simulink model "HybridPowertrain_TestBench_Final"  (R2017a)
settings: Solver=ode1  StartTime=0.0  StopTime=1400  FixedStep=0.01  RelTol=1e-3  EnableMultiTasking=on
undefined symbols (not defined in the file): AccActPos, air, Atm_temp, bms_inletair_temp, BMS_IstStrom, bms_maxchargecurrent, bms_maxdischargecurrent, BMS_Notfallkuehlung, BMS_SOC, BrkPdlPos, cal, Cells, Chg, D1_Commanded_Torque, D1_DC_Bus_Voltage, D2_Motor_Speed, D2_Torque_Feedback, DriverControls, EcoCAR3_Lib, Em, EngActStdyStTorq, Engine, EngSpd, env, ESS, fd, g, gb, Gearbox, GearBox, gps_lat, gps_long, Grade, I_loss, IMG, InstFuelConsmpRate, KeyPosition, lib_ESS_plant_V1_2, Loss, max_vehicle_rad_air_flow, mot, mph2kph, mph2ms, NeutralGear, ParkGear, PPEI_Engine_General_Status_2__ThrPos, PTEI_Engine_Torque_Status__EngActStdyStTorq, R_0, R_1, Ratio, RegenBrkDisable, rho, SampleTime, ShiftLeverPosition, SOC_bp, SOC_init, Spd, Speed, SW_CS_ON, SW_Engine_ON ... (+15)
libraries: simulink x39, fl_lib x13, nesl_utility x8, Utility x1, EC2_libraries x1
(part 1 of 5)
settings Model: Creator=Sajjan  LastModifiedBy=vraj
settings SolverCC: ZeroCrossAlgorithm=Adaptive
settings DataIOCC: LimitDataPoints=on  SaveFormat=Array
settings OptimizationCC: LifeSpan=inf
settings DebuggingCC: SFUnexpectedBacktrackingDiag=warning  SFNoUnconditionalDefaultTransitionDiag=warning  SFExecutionAtInitializationDiag=none
settings HardwareCC: ProdBitPerPointer=32  ProdBitPerSizeT=32  ProdBitPerPtrDiffT=32  ProdLargestAtomicFloat=None  ProdIntDivRoundTo=Undefined  ProdEndianess=Unspecified  ProdWordSize=32  ProdHWDeviceType=32-bit Generic
settings ModelReferenceCC: PropagateSignalLabelsOutOfModel=off
settings GRTTargetCC: TargetLangStandard=C89/C90 (ANSI)  GeneratePreprocessorConditionals=Disable all
settings ConfigComp: CovMetricSettings=dw  CovHtmlReporting=on  CovSaveCumulativeToWorkspaceVar=on  CovSaveSingleToWorkspaceVar=on  CovExternalEMLEnable=off

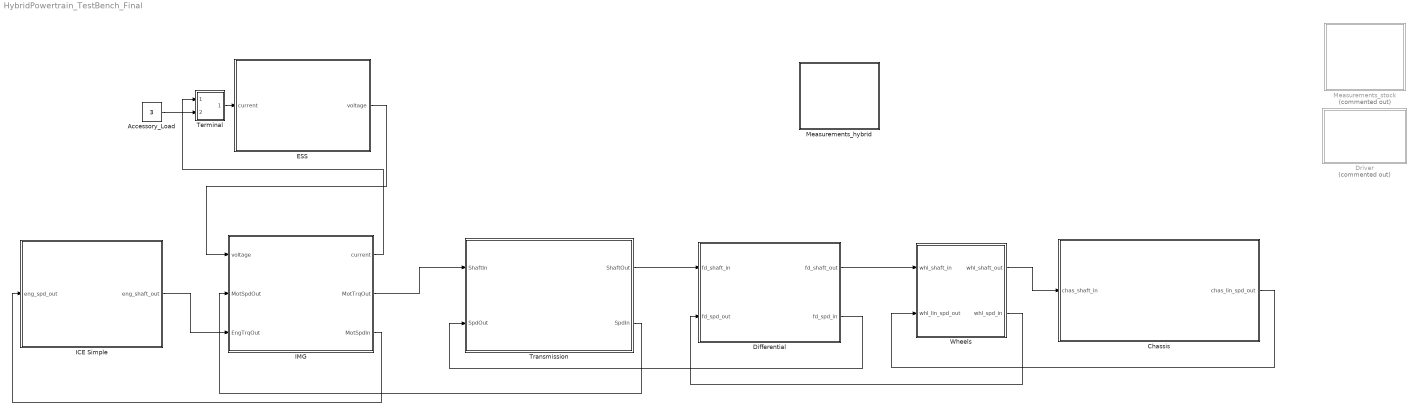
== system HybridPowertrain_TestBench_Final ==
  Accessory_Load : Constant  Value=3
  Chassis : Subsystem  AncestorBlock=Chassis/Chassis
      mask Display:
      | image('/media/vraj/Matlab/Workspace/EcoCAR3/MIL_Code/P2_PHEV_MIL_EC3Y4_V1/Images/Chassis.JPG');
      | color('red');
      | port_label('input',1,'ShaftIn');
      | port_label('output',1,'SpdOut');
  Differential : Subsystem  AncestorBlock=Differential/Differential
      mask Display:
      | image('Images/Diff.jpg');
      | color('red');
      | port_label('input',1,'ShaftIn')
      | port_label('input',2,'SpdOut')
      | port_label('output',1,'ShaftOut')
      | port_label('output',2,'SpdIn')
  Driver : Subsystem  Commented=on
      mask Display: image('Images\Driver.jpg')
  ESS : Subsystem  AncestorBlock=lib_ESS_plant_V1_2/ESS
      mask Display:
      | image('/media/vraj/Matlab/Workspace/EcoCAR3/MIL_Code/P2_PHEV_MIL_EC3Y4_V1/Images/ESS.jpg')
      | color('red');
      | port_label('Input',1,'Crr');
      | port_label('Output',1,'Volt');
  ICE Simple : Subsystem  AncestorBlock=Engine_simple/ICE Simple
      mask Display:
      | image(imread('EngineTopLevel.jpg'),'center')
      | color('red');
      | port_label('input',1,'SpdOut')
      | port_label('output',1,'ShaftOut')
  IMG : Subsystem  AncestorBlock=IMG/IMG
      mask Display:
      | image(imread('motor.png'),'center')
      | color('red');
      | port_label('Input',1,'Volt');
      | port_label('Input',2,'MotSpdOut');
      | port_label('Output',1,'Crr');
      | port_label('Output',2,'MotTrqOut');
      | port_label('Output',3,'MotSpdIn');
  Measurements_hybrid : Subsystem
  Measurements_stock : Subsystem  Commented=on
  Terminal : Subsystem
  Transmission : Subsystem  AncestorBlock=Transmission/Transmission
      mask Display:
      | image('/media/vraj/Matlab/Workspace/EcoCAR3/MIL_Code/P2_PHEV_MIL_EC3Y4_V1/Images/Trans.PNG')
      | color('red');
      | port_label('Input',1,'ShaftIn')
      | port_label('Input',2,'SpdOut')
      | port_label('Output',1,'ShaftOut')
      | port_label('Output',2,'SpdIn')
  Wheels : Subsystem  AncestorBlock=Wheels/Wheels
      mask Display:
      | image('Images/Wheel.jpg');
      | color('red');
      | port_label('input',1,'ShaftIn');
      | port_label('input',2,'SpdOut');
      | port_label('output',1,'ShaftOut');
      | port_label('output',2,'SpdIn');
  wires:
  Differential/1(fd_shaft_out) -> Wheels/1(whl_shaft_in)
  Wheels/1(whl_shaft_out) -> Chassis/1(chas_shaft_in)
  Chassis/1(chas_lin_spd_out) -> Wheels/2(whl_lin_spd_out)
  Differential/2(fd_spd_in) -> Transmission/2(SpdOut)
  Transmission/1(ShaftOut) -> Differential/1(fd_shaft_in)
  Transmission/2(SpdIn) -> IMG/2(MotSpdOut)
  Wheels/2(whl_spd_in) -> Differential/2(fd_spd_out)
  IMG/3(MotSpdIn) -> ICE Simple/1(eng_spd_out)
  ESS/1(voltage) -> IMG/1(voltage)
  Terminal/1(Out1) -> ESS/1(current)
  Accessory_Load/1 -> Terminal/2(In2)
  IMG/2(MotTrqOut) -> Transmission/1(ShaftIn)
  ICE Simple/1(eng_shaft_out) -> IMG/3(EngTrqOut)
  IMG/1(current) -> Terminal/1(In1)

== system HybridPowertrain_TestBench_Final/Chassis ==
  note: Total opposing
      | force (N)
  chas_shaft_in : Inport
  >1 : Saturate  UpperLimit=inf  LowerLimit=0
  Bus Selector : BusSelector  OutputSignals=veh_grade_force_simu,drag force
  Bus Selector1 : BusSelector  OutputSignals=whl_force_out_simu,whl_mass_out_simu
  Clock : Clock
  Driver Interface : Subsystem
  Grade : Lookup  InputValues=time  Table=Grade
  Soft BCM : Subsystem
      mask Display: image('SoftECU.jpg')
  Sum2 : Sum  Inputs=|++  SaturateOnIntegerOverflow=on  InputSameDT=on  OutDataTypeStr=Inherit: Same as first input
  Sum3 : Sum  Inputs=-+  SaturateOnIntegerOverflow=on  InputSameDT=on  OutDataTypeStr=Inherit: Same as first input
  To Workspace1 : ToWorkspace  VariableName=distance_miles_hist  SampleTime=-1
      settings: Decimation=WORKSPACE_DECIMATION
  To Workspace2 : ToWorkspace  VariableName=veh_dist_meter_hist  SampleTime=-1
      settings: Decimation=WORKSPACE_DECIMATION
  To Workspace3 : ToWorkspace  VariableName=veh_spd_mps_hist  SampleTime=-1
      settings: Decimation=WORKSPACE_DECIMATION
  To Workspace7 : ToWorkspace  VariableName=veh_spd_mph_hist  SampleTime=-1
      settings: Decimation=WORKSPACE_DECIMATION
  Velocity1 : Integrator  LimitOutput=on  LowerSaturationLimit=0
  Velocity2 : Integrator  LimitOutput=on  LowerSaturationLimit=0
  m to miles : Gain  Gain=0.00062
  m to miles1 : Gain  Gain=1/1000
  m/s to kph : Gain  Gain=3.6
  ms to mph : Gain  Gain=1/mph2ms
  non-zero division1 : Subsystem
      mask Display: disp('divider \n I1/I2')
  vehicle losses : Subsystem
  vehicle total mass : Constant  Value=veh.init.mass
  chas_lin_spd_out : Outport
  tag scope: BCM_to_HCU=global, chas_plant_force_in=global, chas_plant_force_loss=global, chas_plant_grade=global, chas_plant_lin_accel=global, chas_plant_lin_spd_out=global, chas_plant_mass=global, chas_plant_mass_static=global, veh_dist_km=global, veh_dist_miles=global
  wires:
  Grade/1 -> vehicle losses/2(Road grade), [chas_plant_grade]
  Bus Selector/2 -> [chas_plant_force_loss]  "<drag force>"
  Bus Selector/1 -> [chas_plant_force_grade]  "<veh_grade_force_simu>"
  vehicle total mass/1 -> Sum2/1, [chas_plant_mass_static]
  Velocity1/1 -> vehicle losses/1(veh spd simu), m/s to kph/1, Velocity2/1, To Workspace3/1, ms to mph/1, chas_lin_spd_out/1
  non-zero division1/1(Out1) -> Velocity1/1, [chas_plant_lin_accel]
  Sum3/1 -> non-zero division1/1(In1)
  Sum2/1 -> non-zero division1/2(In2), [chas_plant_mass]
  >1/1 -> Sum2/2
  Bus Selector1/2 -> >1/1  "<whl_mass_out_simu>"
  Bus Selector1/1 -> [chas_plant_force_in], Sum3/2  "<whl_force_out_simu>"
  chas_shaft_in/1 -> Bus Selector1/1
  vehicle losses/1(info) -> Bus Selector/1
  Soft BCM/1(Out1) -> [BCM_to_HCU]
  m/s to kph/1 -> [chas_plant_lin_spd_out]
  ms to mph/1 -> To Workspace7/1
  Clock/1 -> Grade/1
  Velocity2/1 -> To Workspace2/1, m to miles1/1, m to miles/1
  m to miles/1 -> [veh_dist_miles], To Workspace1/1
  m to miles1/1 -> [veh_dist_km]
  vehicle losses/2(veh_force_loss_simu) -> Sum3/1

== system HybridPowertrain_TestBench_Final/Differential ==
  fd_shaft_in : Inport
  fd_spd_out : Inport  Port=2
  Bus Creator : BusCreator  Inputs=2
  Bus Selector : BusSelector  OutputSignals=gb_trq_out,gb_inertia_out
  Inertia calculation : Subsystem
  Speed calculation : Subsystem
  Torque calculation : Subsystem
  fd_shaft_out : Outport
  fd_spd_in : Outport  Port=2
  wires:
  Torque calculation/1(trq out) -> Bus Creator/1  "fd_trq_out_simu"
  fd_spd_out/1 -> Speed calculation/1(spd out)
  Speed calculation/1(spd in) -> Torque calculation/1(spd in), fd_spd_in/1
  Inertia calculation/1(inertia out) -> Bus Creator/2  "fd_inertia_out_simu"
  Bus Selector/1 -> Torque calculation/2(trq in)  "<gb_trq_out>"
  Bus Selector/2 -> Inertia calculation/1(inertia in)  "<gb_inertia_out>"
  fd_shaft_in/1 -> Bus Selector/1
  Bus Creator/1 -> fd_shaft_out/1

== system HybridPowertrain_TestBench_Final/Driver ==
  Bus Creator : BusCreator  Inputs=10
  Bus Selector : BusSelector  OutputSignals=GFD_Light,HV_Chg_Light,Veh_Ready_Light
  Constant : Constant  Commented=on  Value=0
  Display : Display
  Display1 : Display
  Display2 : Display
  Driver Control : Subsystem
  Manual Control : Subsystem  Commented=on
  Multiport Switch1 : MultiPortSwitch  Commented=on  DataPortOrder=Zero-based contiguous  Inputs=2
  Subsystem : Subsystem
  tag scope: Driver_Request=global
  wires:
  Driver Control/1(Key Position) -> Bus Creator/1  "KeyPos"
  Driver Control/2(APP[%]) -> Subsystem/1(In1)  "drv_APP_req_[%]"
  Driver Control/3(BPP[%]) -> Bus Creator/4  "drv_BPP_req_[%]"
  Driver Control/4(Shift Lever Position) -> Bus Creator/5  "ShiftLvrPos"
  Driver Control/5(EVSE_Pluggin) -> Bus Creator/6  "EVSE_Plugged"
  Constant/1 -> Multiport Switch1/1
  Manual Control/1(Out1) -> Multiport Switch1/3
  Bus Creator/1 -> [Driver_Request]
  Driver Control/6(Veh_Spd) -> Bus Creator/7  "Veh_Spd"
  Driver Control/7(Regen_Disable) -> Bus Creator/8  "SW_Regen_Disable"
  Driver Control/8(Engine_On) -> Bus Creator/9  "SW_Engine_ON"
  Driver Control/9(CS_On) -> Bus Creator/10  "SW_CS_ON"
  [Digital] -> Bus Selector/1
  Bus Selector/1 -> Display/1  "<GFD_Light>"
  Bus Selector/2 -> Display1/1  "<HV_Chg_Light>"
  Bus Selector/3 -> Display2/1  "<Veh_Ready_Light>"
  Subsystem/1(APP1) -> Bus Creator/2
  Subsystem/2(APP2) -> Bus Creator/3

== system HybridPowertrain_TestBench_Final/ESS ==
  note: BMS_to_Actuators
  current : Inport
  ESS : Subsystem
      mask Display:
      | image('/media/vraj/Matlab/Workspace/EcoCAR3/MIL_Code/P2_PHEV_MIL_EC3Y4_V1/Images/ESS.jpg')
      | color('red');
      | port_label('Input',2,'Crr');
      | port_label('Output',2,'Volt');
  Inputs : Subsystem  AncestorBlock=lib_DCDC/DC-DC Converter/Inputs
  Outputs : Subsystem
  Soft BMS : Subsystem  RequirementInfo={} %GIDa_f148d73b_346e_4e28_9569_8b82e4a6609c
      mask Display: image('/media/vraj/Matlab/Workspace/EcoCAR3/MIL_Code/P2_PHEV_MIL_EC3Y4_V1/Images/SoftECU.jpg')
  voltage : Outport
  wires:
  current/1 -> ESS/2("Crr ")
  Soft BMS/2(Output2) -> ESS/1("In ")
  ESS/1(out) -> Soft BMS/2(Input2)  "Sensors_to_BMS"
  ESS/2(Voltage) -> voltage/1
  Soft BMS/1(CAN) -> Outputs/1(Outputs)
  Inputs/1(Inputs) -> Soft BMS/1(Input1)

== system HybridPowertrain_TestBench_Final/ICE Simple ==
  eng_spd_out : Inport
  Engine Plant Modified : Subsystem
      mask Display:
      | image(imread('EngineTopLevel.jpg'),'center')
      | color('red');
      | port_label('input',2,'SpdOut')
      | port_label('output',2,'ShaftOut')
  Inputs : Subsystem
  Soft ECM : Subsystem
      mask Display: image('SoftECU.jpg')
  eng_shaft_out : Outport
  tag scope: ECM_to_HCU=global
  wires:
  Engine Plant Modified/2(eng_shaft_out) -> eng_shaft_out/1
  eng_spd_out/1 -> Engine Plant Modified/2(eng_spd_out)
  Soft ECM/2(Out1) -> Engine Plant Modified/1("In ")  "ECM_to_Actuators"
  Inputs/1(Inputs) -> Soft ECM/1(In)
  Soft ECM/1(Out) -> [ECM_to_HCU]
  Engine Plant Modified/1(Out) -> Soft ECM/2(In1)

== system HybridPowertrain_TestBench_Final/IMG ==
  voltage : Inport
  MotSpdOut : Inport  Port=2
  EngTrqOut : Inport  Port=3
  IMG Plant : Subsystem
      mask Display:
      | image('/media/vraj/Matlab/Workspace/EcoCAR3/MIL_Code/P2_PHEV_MIL_EC3Y4_V1/Images/motor.png')
      | color('red');
      | port_label('Input',2,'Volt');
      | port_label('Input',3,'SpdOut');
      | port_label('Input',1,'MCU_cmd');
      | port_label('Output',1,'Sensor_Out');
      | port_label('Output',2,'Crr');
      | port_label('Output',3,'MotTrqOut');
      | port_label('Output',4,'MotSpdIn');
  Soft MCU : Subsystem
      mask Display: image('/media/vraj/Matlab/Workspace/EcoCAR3/MIL_Code/P2_PHEV_MIL_EC3Y4_V1/Images/SoftECU.jpg')
  current : Outport
  MotTrqOut : Outport  Port=2
  MotSpdIn : Outport  Port=3
  tag scope: MCU_to_HCU=global
  wires:
  IMG Plant/1(Out1) -> Soft MCU/2(In1)  "Sensors_to_MCU"
  Soft MCU/2(Out1) -> IMG Plant/1("In1 ")  "MCU_to_Actuators"
  Soft MCU/1(Out) -> [MCU_to_HCU]
  [HCU_to_HV_CAN] -> Soft MCU/1(In)
  IMG Plant/2(current) -> current/1
  voltage/1 -> IMG Plant/2(voltage)
  IMG Plant/3(MotTrqOut) -> MotTrqOut/1
  MotSpdOut/1 -> IMG Plant/3(SpdOut)
  IMG Plant/4(MotSpdIn) -> MotSpdIn/1
  EngTrqOut/1 -> IMG Plant/4(EngTrqOut)

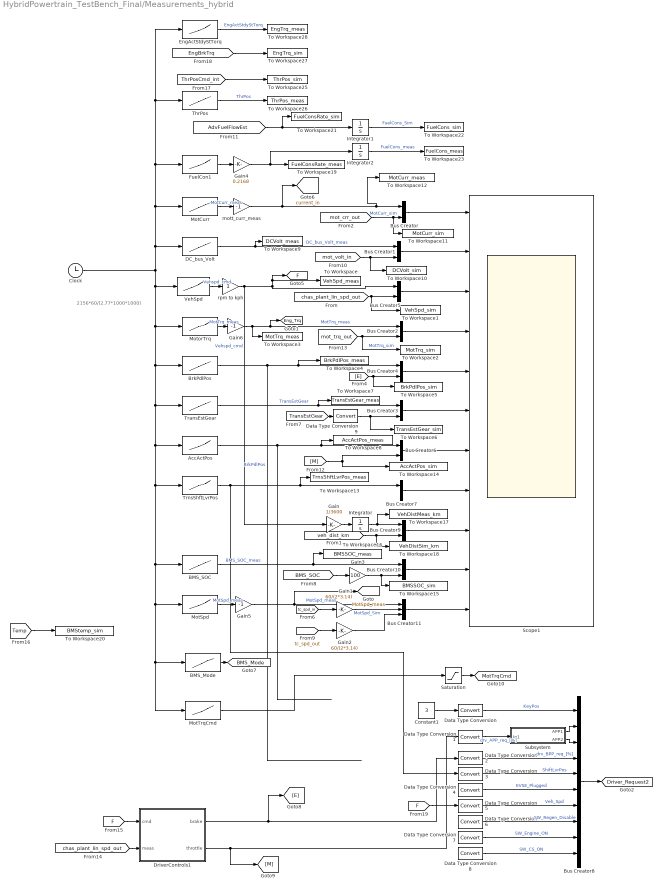
== system HybridPowertrain_TestBench_Final/Measurements_hybrid ==
  note: 2156*60/(2.77*1000*1000)
  AccActPos : Lookup  InputValues=Times  Table=AccActPos
  BMS_Mode : Lookup  InputValues=[0 0.9 1 2 3]  Table=[0 0 1 1 1]
  BMS_SOC : Lookup  InputValues=Times  Table=BMS_SOC
  BrkPdlPos : Lookup  InputValues=Times  Table=BrkPdlPos
  Bus Creator{,1..7,9..10} (10 alike) : BusCreator  Inputs=2
  Bus Creator11 : BusCreator  Inputs=3
  Bus Creator8 : BusCreator  Inputs=10
  Clock : Clock
  Constant1 : Constant  Value=3
  DC_bus_Volt : Lookup  InputValues=Times  Table=D1_DC_Bus_Voltage
  Data Type Conversion{,1..9} (10 alike) : DataTypeConversion
  DriverControls1 : Subsystem  AncestorBlock=EcoCAR3_Lib/DriverControls
  EngActStdyStTorq : Lookup  InputValues=Times  Table=EngActStdyStTorq
  FuelCon1 : Lookup  InputValues=Times  Table=InstFuelConsmpRate
  Gain : Gain  Gain=1/3600
  Gain1 : Gain  Gain=60/(2*3.14)
  Gain2 : Gain  Gain=60/(2*3.14)
  Gain3 : Gain  Gain=100
  Gain4 : Gain  Gain=0.2168
  Gain5 : Gain  Gain=-1
  Gain6 : Gain  Gain=-1
  Integrator : Integrator
  Integrator1 : Integrator
  Integrator2 : Integrator
  MotCurr : Lookup  InputValues=Times  Table=BMS_IstStrom
  MotSpd : Lookup  InputValues=Times  Table=D2_Motor_Speed
  MotTrqCmd : Lookup  InputValues=Times  Table=D1_Commanded_Torque
  MotorTrq : Lookup  InputValues=Times  Table=D2_Torque_Feedback
  Saturation : Saturate  UpperLimit=150  LowerLimit=0
  Scope1 : Scope  NumInputPorts=11
  Subsystem : Subsystem
  ThrPos : Lookup  InputValues=Times  Table=ThrPos
  To Workspace : ToWorkspace  VariableName=VehSpd_meas  SaveFormat=Timeseries  SampleTime=-1
  To Workspace1 : ToWorkspace  VariableName=VehSpd_sim  SaveFormat=Timeseries  SampleTime=-1
  To Workspace10 : ToWorkspace  VariableName=DCVolt_sim  SaveFormat=Timeseries  SampleTime=-1
  To Workspace11 : ToWorkspace  VariableName=MotCurr_sim  SaveFormat=Timeseries  SampleTime=-1
  To Workspace12 : ToWorkspace  VariableName=MotCurr_meas  SaveFormat=Timeseries  SampleTime=-1
  To Workspace13 : ToWorkspace  VariableName=TrnsShftLvrPos_meas  SaveFormat=Timeseries  SampleTime=-1
  To Workspace14 : ToWorkspace  VariableName=AccActPos_sim  SaveFormat=Timeseries  SampleTime=-1
  To Workspace15 : ToWorkspace  VariableName=BMSSOC_sim  SaveFormat=Timeseries  SampleTime=-1
  To Workspace16 : ToWorkspace  VariableName=BMSSOC_meas  SaveFormat=Timeseries  SampleTime=-1
  To Workspace17 : ToWorkspace  VariableName=VehDistMeas_km  SaveFormat=Timeseries  SampleTime=-1
  To Workspace18 : ToWorkspace  VariableName=VehDistSim_km  SaveFormat=Timeseries  SampleTime=-1
  To Workspace19 : ToWorkspace  VariableName=FuelConsRate_meas  SaveFormat=Timeseries  SampleTime=-1
  To Workspace2 : ToWorkspace  VariableName=MotTrq_sim  SaveFormat=Timeseries  SampleTime=-1
  To Workspace20 : ToWorkspace  VariableName=BMStemp_sim  SaveFormat=Timeseries  SampleTime=-1
  To Workspace21 : ToWorkspace  VariableName=FuelConsRate_sim  SaveFormat=Timeseries  SampleTime=-1
  To Workspace22 : ToWorkspace  VariableName=FuelCons_sim  SaveFormat=Timeseries  SampleTime=-1
  To Workspace23 : ToWorkspace  VariableName=FuelCons_meas  SaveFormat=Timeseries  SampleTime=-1
  To Workspace25 : ToWorkspace  VariableName=ThrPos_sim  SaveFormat=Timeseries  SampleTime=-1
  To Workspace26 : ToWorkspace  VariableName=ThrPos_meas  SaveFormat=Timeseries  SampleTime=-1
  To Workspace27 : ToWorkspace  VariableName=EngTrq_sim  SaveFormat=Timeseries  SampleTime=-1
  To Workspace28 : ToWorkspace  VariableName=EngTrq_meas  SaveFormat=Timeseries  SampleTime=-1
  To Workspace3 : ToWorkspace  VariableName=MotTrq_meas  SaveFormat=Timeseries  SampleTime=-1
  To Workspace4 : ToWorkspace  VariableName=BrkPdlPos_meas  SaveFormat=Timeseries  SampleTime=-1
  To Workspace5 : ToWorkspace  VariableName=BrkPdlPos_sim  SaveFormat=Timeseries  SampleTime=-1
  To Workspace6 : ToWorkspace  VariableName=TransEstGear_sim  SaveFormat=Timeseries  SampleTime=-1
  To Workspace7 : ToWorkspace  VariableName=TransEstGear_meas  SaveFormat=Timeseries  SampleTime=-1
  To Workspace8 : ToWorkspace  VariableName=AccActPos_meas  SaveFormat=Timeseries  SampleTime=-1
  To Workspace9 : ToWorkspace  VariableName=DCVolt_meas  SaveFormat=Timeseries  SampleTime=-1
  TransEstGear : Lookup  InputValues=Times  Table=TransEstGear
  TrnsShftLvrPos : Lookup  InputValues=Times  Table=TrnsShftLvrPos
  VehSpd : Lookup_n-D  NumberOfTableDimensions=1  BreakpointsForDimension1=Times  Table=WhlGrndVlctyRtDrvn  InternalRulePriority=Speed  RndMeth=Simplest  InputSameDT=on
  mott_curr_meas : Gain  Gain=-1
  rpm to kph : Gain
  tag scope: BMS_Mode=global, Driver_Request2=global, Eng_Trq=global, F=global, MotSpd_meas=global, MotTrqCmd=global, current_in=global
  wires:
  Gain2/1 -> Bus Creator11/3
  [tc_spd_out] -> Gain2/1
  Gain1/1 -> Bus Creator11/2  "MotSpd_Sim"
  Bus Creator11/1 -> Scope1/11
  [tc_spd_in] -> Gain1/1
  Gain5/1 -> [MotSpd_meas], Bus Creator11/1  "MotSpd_meas"
  Bus Creator10/1 -> Scope1/10
  Gain/1 -> Integrator/1
  Bus Creator9/1 -> Scope1/9
  Integrator/1 -> To Workspace17/1, Bus Creator9/1
  [veh_dist_km] -> Bus Creator9/2, To Workspace18/1
  [M] -> Bus Creator6/2, To Workspace14/1
  Data Type Conversion9/1 -> To Workspace6/1, Bus Creator3/2
  [F] -> Data Type Conversion5/1
  Constant1/1 -> Data Type Conversion/1
  Subsystem/2(APP2) -> Bus Creator8/3
  Subsystem/1(APP1) -> Bus Creator8/2
  Data Type Conversion8/1 -> Bus Creator8/10  "SW_CS_ON"
  Data Type Conversion7/1 -> Bus Creator8/9  "SW_Engine_ON"
  Data Type Conversion6/1 -> Bus Creator8/8  "SW_Regen_Disable"
  Data Type Conversion5/1 -> Bus Creator8/7  "Veh_Spd"
  Bus Creator8/1 -> [Driver_Request2]
  Data Type Conversion4/1 -> Bus Creator8/6  "EVSE_Plugged"
  Data Type Conversion3/1 -> Bus Creator8/5  "ShiftLvrPos"
  Data Type Conversion2/1 -> Bus Creator8/4  "drv_BPP_req_[%]"
  Data Type Conversion1/1 -> Subsystem/1(In1)  "drv_APP_req_[%]"
  Data Type Conversion/1 -> Bus Creator8/1  "KeyPos"
  Bus Creator7/1 -> Scope1/8
  Bus Creator6/1 -> Scope1/7
  TrnsShftLvrPos/1 -> To Workspace13/1, Bus Creator7/1, Data Type Conversion3/1
  [TransEstGear] -> Data Type Conversion9/1
  Bus Creator4/1 -> Scope1/5
  DC_bus_Volt/1 -> To Workspace9/1, Bus Creator1/1  "DC_bus_Volt_meas"
  TransEstGear/1 -> To Workspace7/1, Bus Creator3/1  "TransEstGear"
  Bus Creator1/1 -> Scope1/2
  Bus Creator3/1 -> Scope1/6
  BrkPdlPos/1 -> To Workspace4/1, Bus Creator4/1  "BrkPdlPos"
  Gain6/1 -> [Eng_Trq], Bus Creator2/1, To Workspace3/1  "MotTrq_meas"
  Bus Creator2/1 -> Scope1/4
  Bus Creator/1 -> Scope1/1
  MotCurr/1 -> mott_curr_meas/1  "MotCurr_meas"
  [mot_crr_out] -> To Workspace11/1, Bus Creator/2  "MotCurr_sim"
  [chas_plant_lin_spd_out] -> Bus Creator5/2, To Workspace1/1
  [E] -> Bus Creator4/2, To Workspace5/1
  rpm to kph/1 -> [F], To Workspace/1, Bus Creator5/1, Gain/1  "Vehspd_cmd"
  [mot_trq_out] -> To Workspace2/1, Bus Creator2/2  "MotTrq_sim"
  Bus Creator5/1 -> Scope1/3
  [mot_volt_in] -> To Workspace10/1, Bus Creator1/2
  BMS_SOC/1 -> Bus Creator10/1, To Workspace16/1  "BMS_SOC_meas"
  [BMS_SOC] -> Gain3/1
  BMS_Mode/1 -> [BMS_Mode]
  Gain3/1 -> Bus Creator10/2, To Workspace15/1
  VehSpd/1 -> rpm to kph/1  "Vehspd_cmd"
  DriverControls1/1(brake) -> Data Type Conversion2/1, [E]
  MotSpd/1 -> Gain5/1  "MotSpd_meas"
  MotorTrq/1 -> Gain6/1  "MotTrq_meas"
  [F] -> DriverControls1/1(cmd)
  [chas_plant_lin_spd_out] -> DriverControls1/2(meas)
  DriverControls1/2(throttle) -> Data Type Conversion1/1, [M]
  Saturation/1 -> [MotTrqCmd]
  MotTrqCmd/1 -> Saturation/1
  [Temp] -> To Workspace20/1
  AccActPos/1 -> Bus Creator6/1, To Workspace8/1
  mott_curr_meas/1 -> [current_in], Bus Creator/1, To Workspace12/1
  FuelCon1/1 -> Gain4/1
  Gain4/1 -> Integrator2/1, To Workspace19/1
  [AdvFuelFlowEst] -> Integrator1/1, To Workspace21/1
  Integrator1/1 -> To Workspace22/1  "FuelCons_Sim"
  Integrator2/1 -> To Workspace23/1  "FuelCons_meas"
  [ThrPosCmd_int] -> To Workspace25/1
  ThrPos/1 -> To Workspace26/1  "ThrPos"
  [EngBrkTrq] -> To Workspace27/1
  EngActStdyStTorq/1 -> To Workspace28/1  "EngActStdyStTorq"
  Clock/1 -> MotTrqCmd/1, BMS_Mode/1, MotSpd/1, BMS_SOC/1, TrnsShftLvrPos/1, AccActPos/1, TransEstGear/1, BrkPdlPos/1, MotorTrq/1, VehSpd/1, MotCurr/1, ThrPos/1, EngActStdyStTorq/1, FuelCon1/1, DC_bus_Volt/1

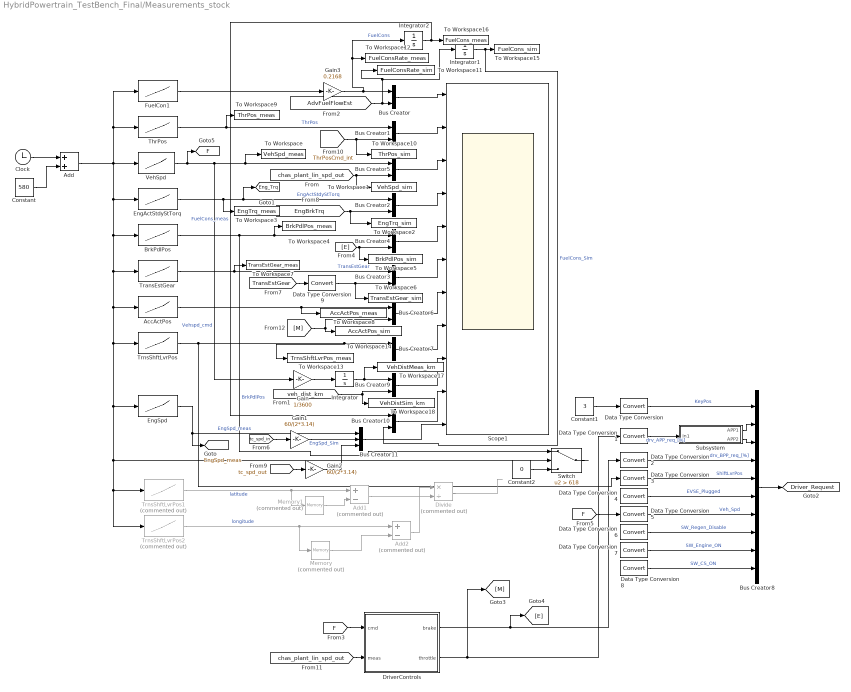
== system HybridPowertrain_TestBench_Final/Measurements_stock ==
  AccActPos : Lookup  InputValues=Time  Table=AccActPos
  Add : Sum
  Add1 : Sum  Commented=on  Inputs=+-
  Add2 : Sum  Commented=on  Inputs=+-
  BrkPdlPos : Lookup  InputValues=Time  Table=BrkPdlPos
  Bus Creator{,1..7,9..10} (10 alike) : BusCreator  Inputs=2
  Bus Creator11 : BusCreator  Inputs=3
  Bus Creator8 : BusCreator  Inputs=10
  Clock : Clock
  Constant : Constant  Value=580
  Constant1 : Constant  Value=3
  Constant2 : Constant  Value=0
  Data Type Conversion{,1..9} (10 alike) : DataTypeConversion
  Divide : Product  Commented=on  Inputs=*/
  DriverControls : Subsystem  AncestorBlock=EcoCAR3_Lib/DriverControls
  EngActStdyStTorq : Lookup  InputValues=Time  Table=PTEI_Engine_Torque_Status__EngActStdyStTorq
  EngSpd : Lookup  InputValues=Time  Table=EngSpd
  FuelCon1 : Lookup  InputValues=Time  Table=InstFuelConsmpRate
  Gain : Gain  Gain=1/3600
  Gain1 : Gain  Gain=60/(2*3.14)
  Gain2 : Gain  Gain=60/(2*3.14)
  Gain3 : Gain  Gain=0.2168
  Integrator : Integrator
  Integrator1 : Integrator
  Integrator2 : Integrator
  Memory : Memory  Commented=on  InheritSampleTime=on
  Memory1 : Memory  Commented=on  InheritSampleTime=on
  Scope1 : Scope  NumInputPorts=11
  Subsystem : Subsystem
  Switch : Switch  Criteria=u2 > Threshold  Threshold=618
  ThrPos : Lookup  InputValues=Time  Table=PPEI_Engine_General_Status_2__ThrPos
  To Workspace : ToWorkspace  VariableName=VehSpd_meas  SaveFormat=Timeseries  SampleTime=-1
  To Workspace1 : ToWorkspace  VariableName=VehSpd_sim  SaveFormat=Timeseries  SampleTime=-1
  To Workspace10 : ToWorkspace  VariableName=ThrPos_sim  SaveFormat=Timeseries  SampleTime=-1
  To Workspace11 : ToWorkspace  VariableName=FuelConsRate_sim  SaveFormat=Timeseries  SampleTime=-1
  To Workspace12 : ToWorkspace  VariableName=FuelConsRate_meas  SaveFormat=Timeseries  SampleTime=-1
  To Workspace13 : ToWorkspace  VariableName=TrnsShftLvrPos_meas  SaveFormat=Timeseries  SampleTime=-1
  To Workspace14 : ToWorkspace  VariableName=AccActPos_sim  SaveFormat=Timeseries  SampleTime=-1
  To Workspace15 : ToWorkspace  VariableName=FuelCons_sim  SaveFormat=Timeseries  SampleTime=-1
  To Workspace16 : ToWorkspace  VariableName=FuelCons_meas  SaveFormat=Timeseries  SampleTime=-1
  To Workspace17 : ToWorkspace  VariableName=VehDistMeas_km  SaveFormat=Timeseries  SampleTime=-1
  To Workspace18 : ToWorkspace  VariableName=VehDistSim_km  SaveFormat=Timeseries  SampleTime=-1
  To Workspace2 : ToWorkspace  VariableName=EngTrq_sim  SaveFormat=Timeseries  SampleTime=-1
  To Workspace3 : ToWorkspace  VariableName=EngTrq_meas  SaveFormat=Timeseries  SampleTime=-1
  To Workspace4 : ToWorkspace  VariableName=BrkPdlPos_meas  SaveFormat=Timeseries  SampleTime=-1
  To Workspace5 : ToWorkspace  VariableName=BrkPdlPos_sim  SaveFormat=Timeseries  SampleTime=-1
  To Workspace6 : ToWorkspace  VariableName=TransEstGear_sim  SaveFormat=Timeseries  SampleTime=-1
  To Workspace7 : ToWorkspace  VariableName=TransEstGear_meas  SaveFormat=Timeseries  SampleTime=-1
  To Workspace8 : ToWorkspace  VariableName=AccActPos_meas  SaveFormat=Timeseries  SampleTime=-1
  To Workspace9 : ToWorkspace  VariableName=ThrPos_meas  SaveFormat=Timeseries  SampleTime=-1
  TransEstGear : Lookup  InputValues=Time  Table=TransEstGear
  TrnsShftLvrPos : Lookup  InputValues=Time  Table=TrnsShftLvrPos
  TrnsShftLvrPos1 : Lookup  Commented=on  InputValues=[0:0.1:3000]  Table=gps_lat
  TrnsShftLvrPos2 : Lookup  Commented=on  InputValues=[0:0.1:3000]  Table=gps_long
  VehSpd : Lookup_n-D  NumberOfTableDimensions=1  BreakpointsForDimension1=Time  Table=VehSpdAvgDrvn  InternalRulePriority=Speed  RndMeth=Simplest  InputSameDT=on
  tag scope: Driver_Request=global, EngSpd_meas=global, Eng_Trq=global, F=global
  wires:
  [ThrPosCmd_int] -> Bus Creator1/2, To Workspace10/1
  Bus Creator5/1 -> Scope1/3
  [EngBrkTrq] -> Bus Creator2/2, To Workspace2/1
  VehSpd/1 -> [F], To Workspace/1, Bus Creator5/1, Gain/1  "Vehspd_cmd"
  [E] -> Bus Creator4/2, To Workspace5/1
  [chas_plant_lin_spd_out] -> To Workspace1/1, Bus Creator5/2
  [AdvFuelFlowEst] -> Integrator1/1, To Workspace11/1, Bus Creator/2
  Gain3/1 -> Integrator2/1, To Workspace12/1, Bus Creator/1  "FuelCons"
  FuelCon1/1 -> Gain3/1
  Bus Creator/1 -> Scope1/1
  Constant/1 -> Add/2
  Bus Creator2/1 -> Scope1/4
  EngActStdyStTorq/1 -> To Workspace3/1, [Eng_Trq], Bus Creator2/1  "EngActStdyStTorq"
  BrkPdlPos/1 -> To Workspace4/1, Bus Creator4/1, Switch/1  "BrkPdlPos"
  Bus Creator3/1 -> Scope1/6
  Bus Creator1/1 -> Scope1/2
  TransEstGear/1 -> To Workspace7/1, Bus Creator3/1  "TransEstGear"
  Clock/1 -> Add/1
  ThrPos/1 -> To Workspace9/1, Bus Creator1/1  "ThrPos"
  Bus Creator4/1 -> Scope1/5
  [TransEstGear] -> Data Type Conversion9/1
  TrnsShftLvrPos/1 -> To Workspace13/1, Bus Creator7/1, Data Type Conversion3/1
  Bus Creator6/1 -> Scope1/7
  Bus Creator7/1 -> Scope1/8
  Data Type Conversion/1 -> Bus Creator8/1  "KeyPos"
  Data Type Conversion1/1 -> Subsystem/1(In1)  "drv_APP_req_[%]"
  Data Type Conversion2/1 -> Bus Creator8/4  "drv_BPP_req_[%]"
  Data Type Conversion3/1 -> Bus Creator8/5  "ShiftLvrPos"
  Data Type Conversion4/1 -> Bus Creator8/6  "EVSE_Plugged"
  Bus Creator8/1 -> [Driver_Request]
  Data Type Conversion5/1 -> Bus Creator8/7  "Veh_Spd"
  Data Type Conversion6/1 -> Bus Creator8/8  "SW_Regen_Disable"
  Data Type Conversion7/1 -> Bus Creator8/9  "SW_Engine_ON"
  Data Type Conversion8/1 -> Bus Creator8/10  "SW_CS_ON"
  Subsystem/1(APP1) -> Bus Creator8/2
  Subsystem/2(APP2) -> Bus Creator8/3
  Constant1/1 -> Data Type Conversion/1
  [F] -> Data Type Conversion5/1
  Data Type Conversion9/1 -> Bus Creator3/2, To Workspace6/1
  AccActPos/1 -> To Workspace8/1, Bus Creator6/1
  [M] -> To Workspace14/1, Bus Creator6/2
  [veh_dist_km] -> To Workspace18/1, Bus Creator9/2
  Integrator/1 -> Bus Creator9/1, To Workspace17/1
  Bus Creator9/1 -> Scope1/9
  Gain/1 -> Integrator/1
  Integrator1/1 -> Bus Creator10/2, To Workspace15/1  "FuelCons_Sim"
  Bus Creator10/1 -> Scope1/10
  Integrator2/1 -> Bus Creator10/1, To Workspace16/1  "FuelCons_meas"
  Switch/1 -> ?
  Add/1 -> EngSpd/1, TrnsShftLvrPos2/1, TrnsShftLvrPos1/1, Switch/2, TrnsShftLvrPos/1, AccActPos/1, TransEstGear/1, BrkPdlPos/1, EngActStdyStTorq/1, FuelCon1/1, ThrPos/1, VehSpd/1
  Constant2/1 -> Switch/3
  TrnsShftLvrPos1/1 -> Add1/1, Memory1/1  "latitude"
  TrnsShftLvrPos2/1 -> Add2/1, Memory/1  "longitude"
  Memory/1 -> Add2/2
  Add2/1 -> Divide/1
  Memory1/1 -> Add1/2
  Add1/1 -> Divide/2
  Divide/1 -> ?
  EngSpd/1 -> Bus Creator11/1, [EngSpd_meas]  "EngSpd_meas"
  [tc_spd_in] -> Gain1/1
  Bus Creator11/1 -> Scope1/11
  Gain1/1 -> Bus Creator11/2  "EngSpd_Sim"
  [tc_spd_out] -> Gain2/1
  Gain2/1 -> Bus Creator11/3
  [F] -> DriverControls/1(cmd)
  [chas_plant_lin_spd_out] -> DriverControls/2(meas)
  DriverControls/1(brake) -> [E], Data Type Conversion2/1
  DriverControls/2(throttle) -> Data Type Conversion1/1, [M]

== system HybridPowertrain_TestBench_Final/Terminal ==
  In1 : Inport
  In2 : Inport  Port=2
  Sum : Sum  Inputs=|++
  Out1 : Outport
  wires:
  In1/1 -> Sum/1
  In2/1 -> Sum/2
  Sum/1 -> Out1/1

== system HybridPowertrain_TestBench_Final/Transmission ==
  ShaftIn : Inport
  SpdOut : Inport  Port=2
  Inputs : Subsystem  AncestorBlock=lib_DCDC/DC-DC Converter/Inputs
  Outputs : Subsystem  AncestorBlock=lib_DCDC/DC-DC Converter/Outputs
  Soft TCM : Subsystem
      mask Display: image('/media/vraj/Matlab/Workspace/EcoCAR3/MIL_Code/P2_PHEV_MIL_EC3Y4_V1/Images/SoftECU.jpg')
  Transmission Plant : Subsystem
      mask Display:
      | image('/media/vraj/Matlab/Workspace/EcoCAR3/MIL_Code/P2_PHEV_MIL_EC3Y4_V1/Images/Trans.PNG')
      | color('red');
      | port_label('Input',2,'ShaftIn')
      | port_label('Input',3,'SpdOut')
      | port_label('Output',2,'ShaftOut')
      | port_label('Output',3,'SpdIn')
  ShaftOut : Outport
  SpdIn : Outport  Port=2
  wires:
  Transmission Plant/3(TorqConvSpdIn) -> SpdIn/1
  Transmission Plant/2(GearboxShaftOut) -> ShaftOut/1
  SpdOut/1 -> Transmission Plant/3(GearboxSpdOut)
  ShaftIn/1 -> Transmission Plant/2(TorqConvShaftIn)
  Soft TCM/1(Out) -> Outputs/1(Outputs)
  Inputs/1(Inputs) -> Soft TCM/1(In)
  Transmission Plant/1(Out1) -> Soft TCM/2(In1)  "Sensors_to_TCM"
  Soft TCM/2(Out1) -> Transmission Plant/1("In1 ")  "TCM_to_Actuators"

== system HybridPowertrain_TestBench_Final/Wheels ==
  whl_shaft_in : Inport
  whl_lin_spd_out : Inport  Port=2
  "1\\radius " : Gain  Gain=1/whl.plant.init.radius  SaturateOnIntegerOverflow=on  OutDataTypeStr=Inherit: Same as input  ParamDataTypeStr=Inherit: Same as input
  Bus Creator : BusCreator  Inputs=2
  Bus Selector : BusSelector  OutputSignals=drv_BPP_req_[%]
  Bus Selector1 : BusSelector  OutputSignals=fd_trq_out_simu,fd_inertia_out_simu
  Clock : Clock
  Force calculation : Subsystem
  Grade : Lookup  InputValues=time  Table=Grade
  Mass calculation : Subsystem
  Speed calculation : Subsystem
  whl_shaft_out : Outport
  whl_spd_in : Outport  Port=2
  wires:
  Bus Selector/1 -> Force calculation/2(BPP[%])  "<drv_BPP_req_[%]>"
  [Driver_Request2] -> Bus Selector/1
  "1\\radius "/1 -> Speed calculation/1(chas_spd)
  Force calculation/1(force) -> Bus Creator/1  "whl_force_out_simu"
  Speed calculation/1(spd in) -> Force calculation/1(spd in), whl_spd_in/1
  Mass calculation/1(Mass) -> Bus Creator/2  "whl_mass_out_simu"
  Bus Selector1/1 -> Force calculation/5(trq_in)  "<fd_trq_out_simu>"
  Bus Selector1/2 -> Force calculation/6(Inertia_In), Mass calculation/1(inertia in)  "<fd_inertia_out_simu>"
  whl_lin_spd_out/1 -> "1\\radius "/1, Force calculation/3(whl_spd)
  whl_shaft_in/1 -> Bus Selector1/1
  Bus Creator/1 -> whl_shaft_out/1
  Grade/1 -> Force calculation/4(grade)
  Clock/1 -> Grade/1

== system HybridPowertrain_TestBench_Final/Chassis/Driver Interface ==
  Bus Selector1 : BusSelector  OutputSignals=KeyPos,drv_APP1,drv_BPP_req_[%],ShiftLvrPos,EVSE_Plugged
  tag scope: EVSEPlugged=global, KeyPosition=global, ShftLvrPos=global, drv_APP_percent2=global, drv_APP_percent=global, drv_BPP_percent=global
  wires:
  Bus Selector1/1 -> [KeyPosition]  "<KeyPos>"
  Bus Selector1/2 -> [drv_APP_percent], [drv_APP_percent2]  "<drv_APP1>"
  Bus Selector1/4 -> [ShftLvrPos]  "<ShiftLvrPos>"
  [Driver_Request2] -> Bus Selector1/1
  Bus Selector1/3 -> [drv_BPP_percent]  "<drv_BPP_req_[%]>"
  Bus Selector1/5 -> [EVSEPlugged]  "<EVSE_Plugged>"

== system HybridPowertrain_TestBench_Final/Chassis/Soft BCM ==
  note: This signal will go to ECM to be transmitted out
      | in the CAN message of PPEI_Vehicle_Speed_and_Distance
  note: Key Position information is collected by BCM and then sent out to HCU by BCM
      | in the CAN message of PPEI_Platforma_General_Status
  Bus Creator : BusCreator  Inputs=2
  Constant : Constant  Value=2
  Data Type Conversion1 : DataTypeConversion
  Data Type Conversion2 : DataTypeConversion
  Data Type Conversion3 : DataTypeConversion
  Data Type Conversion4 : DataTypeConversion  OutDataTypeStr=int8
  Sum : Sum  Inputs=|++
  Switch : Switch  Threshold=1
  Out1 : Outport
  tag scope: VehSpdAvgDrvn=global
  wires:
  [chas_plant_lin_spd_out] -> Data Type Conversion1/1
  Data Type Conversion1/1 -> [VehSpdAvgDrvn]
  [KeyPosition] -> Data Type Conversion2/1
  Data Type Conversion2/1 -> Switch/3, Sum/2  "SysPwrMd"
  Bus Creator/1 -> Out1/1  "BCM_CAN"
  [drv_BPP_percent] -> Data Type Conversion3/1
  Data Type Conversion3/1 -> Bus Creator/2  "BrkPdlPos"
  [KeyPos_Flt_ON] -> Switch/2
  Sum/1 -> Switch/1
  Switch/1 -> Bus Creator/1  "SysPwrMd"
  Constant/1 -> Data Type Conversion4/1
  Data Type Conversion4/1 -> Sum/1

== system HybridPowertrain_TestBench_Final/Chassis/non-zero division1 ==
  note: and finally, the expression is: (u[1] \ u[2]) * 1 = u[1] \ u[2]
  note: (u[2]!=0) is true then returns 1
  note: if u[2] != 0, then output == u[1]\u[2]:
  note: (u[2]==0) is false then returns 0, thus (u[2]+(u[2]==0)) is equal to u[2]+0=u[2]
  note: and finally, the expression is: (u[1] \ 1) * 0 = 0
  note: (u[2]!=0) is false then returns 0
  note: if u[2] == 0, then output == 0:
  note: (u[2]==0) is true then returns 1, thus (u[2]+(u[2]==0)) is equal to 0+1=1
  In1 : Inport
  In2 : Inport  Port=2
  Fcn : Fcn  Expr=u[1]/(u[2]+(u[2]==0))*(u[2]!=0)
  Mux : Mux  Inputs=2
  Out1 : Outport
  wires:
  In2/1 -> Mux/2
  Fcn/1 -> Out1/1
  In1/1 -> Mux/1
  Mux/1 -> Fcn/1

== system HybridPowertrain_TestBench_Final/Chassis/vehicle losses ==
  note: chas.plant.init.mass.body
  veh spd simu : Inport
  Road grade : Inport  Port=2
  Bus Creator : BusCreator  Inputs=2
  Drag Force Calculation : Product  Inputs=6  SaturateOnIntegerOverflow=on  InputSameDT=on  OutDataTypeStr=Inherit: Same as first input
  Grade Force Calculation : Product  Inputs=3  SaturateOnIntegerOverflow=on  InputSameDT=on  OutDataTypeStr=Inherit: Same as first input
  Product1 : Product  SaturateOnIntegerOverflow=on  InputSameDT=on  OutDataTypeStr=Inherit: Same as first input
  Sign : Signum
  Sum3 : Sum  Inputs=|++  SaturateOnIntegerOverflow=on  InputSameDT=on  OutDataTypeStr=Inherit: Same as first input
  Trigonometric Function : Trigonometry
  f1 : Constant  Value=rho
  f2 : Constant  Value=0.5
  f4 : Constant  Value=g
  mass : Constant  Value=1750
  mass1 : Constant  Value=Vehicle.FrontalArea
  mass2 : Constant  Value=Vehicle.Drag
  info : Outport
  veh_force_loss_simu : Outport  Port=2
  wires:
  Bus Creator/1 -> info/1
  Sum3/1 -> veh_force_loss_simu/1  "veh_drag_and_Rx_simu"
  Grade Force Calculation/1 -> Bus Creator/1, Sum3/1  "veh_grade_force_simu"
  veh spd simu/1 -> Sign/1, Drag Force Calculation/2, Drag Force Calculation/1
  Drag Force Calculation/1 -> Product1/2, Bus Creator/2  "drag force"
  Road grade/1 -> Trigonometric Function/1
  Sign/1 -> Product1/1
  Product1/1 -> Sum3/2
  mass/1 -> Grade Force Calculation/1
  f4/1 -> Grade Force Calculation/2
  Trigonometric Function/1 -> Grade Force Calculation/3
  f1/1 -> Drag Force Calculation/4
  mass1/1 -> Drag Force Calculation/5
  f2/1 -> Drag Force Calculation/3
  mass2/1 -> Drag Force Calculation/6

== system HybridPowertrain_TestBench_Final/Differential/Inertia calculation ==
  inertia in : Inport
  Final Drive inertia : Constant  Value=0.02
  Sum3 : Sum  Inputs=|++  SaturateOnIntegerOverflow=on  InputSameDT=on  OutDataTypeStr=Inherit: Same as first input
  "fd.plant.init.ratio " : Gain  Gain=GearBox.L45.FinalDriveRatio  SaturateOnIntegerOverflow=on  OutDataTypeStr=Inherit: Same as input  ParamDataTypeStr=Inherit: Same as input
  inertia out : Outport
  wires:
  "fd.plant.init.ratio "/1 -> Sum3/1
  Final Drive inertia/1 -> Sum3/2
  Sum3/1 -> inertia out/1
  inertia in/1 -> "fd.plant.init.ratio "/1

== system HybridPowertrain_TestBench_Final/Differential/Speed calculation ==
  spd out : Inport
  fd.plant.init.ratio : Gain  Gain=GearBox.L45.FinalDriveRatio  SaturateOnIntegerOverflow=on  OutDataTypeStr=Inherit: Same as input  ParamDataTypeStr=Inherit: Same as input
  spd in : Outport
  wires:
  spd out/1 -> fd.plant.init.ratio/1
  fd.plant.init.ratio/1 -> spd in/1

== system HybridPowertrain_TestBench_Final/Differential/Torque calculation ==
  spd in : Inport
  trq in : Inport  Port=2
  Abs : Abs  SaturateOnIntegerOverflow=on
  Abs1 : Abs  SaturateOnIntegerOverflow=on
  Blending (state dependent) : Subsystem  mask(State dependent blending){xl=-fd.plant.init.spd_thresh, yl=-1, xc=0, yc=0, xr=fd.plant.init.spd_thresh, yr=1}
      mask prompts: xl "Left point (x):"; yl "Left point (y):"; xc "Center point (x):"; yc "Center point (y):"; xr "Right point (x):"; yr "Right point (y):"
      mask help: This block implements state dependent smoothing/blending. IMPORTANT: See help menu.
      mask Help: The output equals the product of the first input and a "hat" function defined by the three points specified in the dialog box.  The second input forms the argument to the hat function.\n\nIMPORTANT: A divide by zero error will result if first coordinates of the three points specified for the hat function are NOT distinct.
      mask Display: plot([-1 1 3 6 8], [1.5 1.5 0.5 4.0 4.0])
  Look-Up Table (2-D) : Subsystem  mask(Lookup Table (2-D)){x=fd.plant.init.trq_loss.idx1_trq, y=fd.plant.init.trq_loss.idx2_spd, t=fd.plant.init.trq_loss.map}
      mask prompts: x "Row:"; y "Column:"; t "Table:"
      mask help: Performs 2-D linear interpolation of input values using the specified input/output table. Extrapolation is performed outside the table boundaries.
      mask init:
      | [r,c]=size(t);
      | xt=reshape(x,prod(size(x)),1);
      | xi=xt(:,ones(1,c));
      | minx=min(x); maxx=max(x);
      | mint=min(min(t)); maxt=max(max(t));
      mask Display: plot(xi,t,[minx maxx],[mint mint],[minx minx],[mint maxt])
  Scope : Scope  NumInputPorts=3
  Sum2 : Sum  Inputs=|+-  SaturateOnIntegerOverflow=on  InputSameDT=on  OutDataTypeStr=Inherit: Same as first input
  fd.plant.init.ratio : Gain  Gain=GearBox.L45.FinalDriveRatio  SaturateOnIntegerOverflow=on  OutDataTypeStr=Inherit: Same as input  ParamDataTypeStr=Inherit: Same as input
  trq out : Outport
  wires:
  Abs/1 -> Look-Up Table (2-D)/1(Rows)
  Abs1/1 -> Look-Up Table (2-D)/2(Cols)
  Look-Up Table (2-D)/1(Out1) -> Blending (state dependent)/1(Input)
  Blending (state dependent)/1(Output) -> Sum2/2, Scope/2
  trq in/1 -> Abs/1, Scope/1, Sum2/1
  Sum2/1 -> fd.plant.init.ratio/1
  fd.plant.init.ratio/1 -> trq out/1
  spd in/1 -> Abs1/1, Scope/3, Blending (state dependent)/2(Control (state))

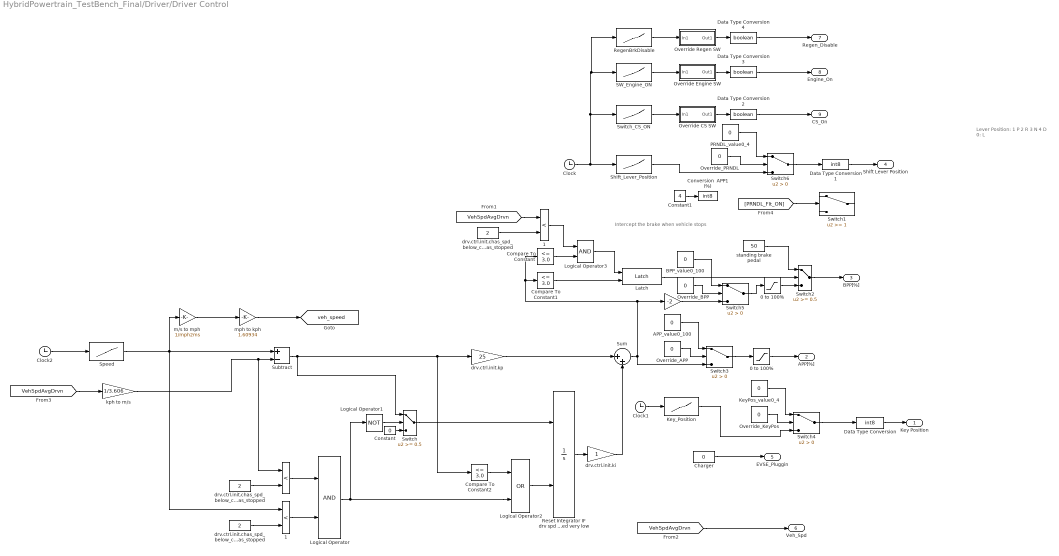
== system HybridPowertrain_TestBench_Final/Driver/Driver Control ==
  note: Lever Position:
      | 1 P
      | 2 R
      | 3 N
      | 4 D
      | 0: L
  note: Intercept the brake when vehicle stops
  " " : Gain  Gain=-2
  "    " : RelationalOperator  Operator=<  RndMeth=Nearest  InputSameDT=on
  "    1" : RelationalOperator  Operator=<  RndMeth=Nearest  InputSameDT=on
  "  1" : RelationalOperator  Operator=<  RndMeth=Nearest  InputSameDT=on
  0 to 100% : Saturate  UpperLimit=100  LowerLimit=0
  "0 to 100% " : Saturate  UpperLimit=100  LowerLimit=0
  APP_value0_100 : Constant  Value=0
  BPP_value0_100 : Constant  Value=0
  Charger : Constant  Value=0
  Clock : Clock
  Clock1 : Clock
  Clock2 : Clock
  Compare To Constant : simulink/Logic and Bit Operations/Compare To Constant  relop=<=  const=3.0  OutDataTypeStr=boolean
  Compare To Constant1 : simulink/Logic and Bit Operations/Compare To Constant  relop=<=  const=3.0  OutDataTypeStr=boolean
  Compare To Constant2 : simulink/Logic and Bit Operations/Compare To Constant  relop=<=  const=3.0  OutDataTypeStr=boolean
  Constant : Constant  Value=0
  Constant1 : Constant  Value=4
  Conversion  APP1 (%) : DataTypeConversion  OutDataTypeStr=int8
  Data Type Conversion : DataTypeConversion  OutDataTypeStr=int8
  Data Type Conversion1 : DataTypeConversion  OutDataTypeStr=int8
  Data Type Conversion2 : DataTypeConversion  OutDataTypeStr=boolean
  Data Type Conversion3 : DataTypeConversion  OutDataTypeStr=boolean
  Data Type Conversion4 : DataTypeConversion  OutDataTypeStr=boolean
  KeyPos_value0_4 : Constant  Value=0
  Key_Position : Lookup  InputValues=time  Table=KeyPosition
  Latch : Utility/Latch
  Logical Operator : Logic  AllPortsSameDT=off  OutDataTypeStr=boolean
  Logical Operator1 : Logic  Operator=NOT  AllPortsSameDT=off  OutDataTypeStr=boolean
  Logical Operator2 : Logic  Operator=OR  AllPortsSameDT=off  OutDataTypeStr=boolean
  Logical Operator3 : Logic  AllPortsSameDT=off  OutDataTypeStr=boolean
  Override CS SW : Subsystem
  Override Engine SW : Subsystem
  Override Regen SW : Subsystem
  Override_APP : Constant  Value=0
  Override_BPP : Constant  Value=0
  Override_KeyPos : Constant  Value=0
  Override_PRNDL : Constant  Value=0
  PRNDL_value0_4 : Constant  Value=0
  RegenBrkDisable : Lookup  InputValues=time  Table=RegenBrkDisable
  Reset Integrator IF drv spd dmd very low AND AND current vehicle speed very low : Integrator  ExternalReset=either
  SW_Engine_ON : Lookup  InputValues=time  Table=SW_Engine_ON
  Shift_Lever_Position : Lookup  InputValues=time  Table=ShiftLeverPosition
  Speed : Lookup  InputValues=time  Table=Speed
  Subtract : Sum  Inputs=+-
  Sum : Sum  Inputs=|++  SaturateOnIntegerOverflow=on  InputSameDT=on  OutDataTypeStr=Inherit: Same as first input
  Switch : Switch  Threshold=0.5
  Switch1 : Switch  Threshold=1
  Switch2 : Switch  Threshold=0.5
  Switch{3..6} (4 alike) : Switch  Criteria=u2 > Threshold
  Switch_CS_ON : Lookup  InputValues=time  Table=SW_CS_ON
  "drv.ctrl.init.chas_spd_below_chas_stopped " : Constant  Value=2
  "drv.ctrl.init.chas_spd_below_chas_stopped " : Constant  Value=2
  "drv.ctrl.init.chas_spd_below_chas_stopped " : Constant  Value=2
  drv.ctrl.init.ki : Gain  SaturateOnIntegerOverflow=on  OutDataTypeStr=Inherit: Same as input  ParamDataTypeStr=Inherit: Same as input
  drv.ctrl.init.kp : Gain  Gain=25  SaturateOnIntegerOverflow=on  OutDataTypeStr=Inherit: Same as input  ParamDataTypeStr=Inherit: Same as input
  kph to m/s : Gain  Gain=1/3.606  SaturateOnIntegerOverflow=on  OutDataTypeStr=Inherit: Same as input  ParamDataTypeStr=Inherit: Same as input
  m/s to mph : Gain  Gain=1/mph2ms
  mph to kph : Gain  Gain=1.60934
  standing brake pedal : Constant  Value=50
  Key Position : Outport
  APP[%] : Outport  Port=2
  BPP[%] : Outport  Port=3
  Shift Lever Position : Outport  Port=4
  EVSE_Pluggin : Outport  Port=5
  Veh_Spd : Outport  Port=6
  Regen_Disable : Outport  Port=7
  Engine_On : Outport  Port=8
  CS_On : Outport  Port=9
  tag scope: veh_speed=global
  wires:
  drv.ctrl.init.kp/1 -> Sum/1
  "    "/1 -> Logical Operator/1
  Speed/1 -> Subtract/1, m/s to mph/1, "  1"/1
  Constant/1 -> Switch/3
  Reset Integrator IF drv spd dmd very low AND AND current vehicle speed very low/1 -> drv.ctrl.init.ki/1
  kph to m/s/1 -> Subtract/2, "    "/1
  Logical Operator1/1 -> Switch/2
  "drv.ctrl.init.chas_spd_below_chas_stopped "/1 -> "    "/2
  Switch/1 -> Reset Integrator IF drv spd dmd very low AND AND current vehicle speed very low/1
  Logical Operator2/1 -> Reset Integrator IF drv spd dmd very low AND AND current vehicle speed very low/2
  "drv.ctrl.init.chas_spd_below_chas_stopped "/1 -> "  1"/2
  drv.ctrl.init.ki/1 -> Sum/2
  "  1"/1 -> Logical Operator/2
  Logical Operator/1 -> Logical Operator2/2, Logical Operator1/1
  "0 to 100% "/1 -> Switch2/3
  " "/1 -> Switch5/3
  [VehSpdAvgDrvn] -> kph to m/s/1
  standing brake pedal/1 -> Switch2/1
  Switch2/1 -> BPP[%]/1
  [VehSpdAvgDrvn] -> "    1"/1
  "drv.ctrl.init.chas_spd_below_chas_stopped "/1 -> "    1"/2
  "    1"/1 -> Logical Operator3/1
  Sum/1 -> Compare To Constant1/1, Compare To Constant/1, " "/1, Switch3/3
  Logical Operator3/1 -> Latch/1
  Compare To Constant/1 -> Logical Operator3/2
  Compare To Constant1/1 -> Latch/2
  Shift_Lever_Position/1 -> Switch6/3
  Data Type Conversion/1 -> Key Position/1
  Data Type Conversion1/1 -> Shift Lever Position/1
  Charger/1 -> EVSE_Pluggin/1
  Subtract/1 -> Compare To Constant2/1, drv.ctrl.init.kp/1, Switch/1
  Compare To Constant2/1 -> Logical Operator2/1
  Clock/1 -> RegenBrkDisable/1, SW_Engine_ON/1, Switch_CS_ON/1, Shift_Lever_Position/1
  Clock1/1 -> Key_Position/1
  Clock2/1 -> Speed/1
  m/s to mph/1 -> mph to kph/1
  mph to kph/1 -> [veh_speed]
  0 to 100%/1 -> APP[%]/1
  Switch_CS_ON/1 -> Override CS SW/1(In1)
  SW_Engine_ON/1 -> Override Engine SW/1(In1)
  RegenBrkDisable/1 -> Override Regen SW/1(In1)
  Override Regen SW/1(Out1) -> Data Type Conversion4/1
  Override Engine SW/1(Out1) -> Data Type Conversion3/1
  Override CS SW/1(Out1) -> Data Type Conversion2/1
  Data Type Conversion2/1 -> CS_On/1
  Data Type Conversion4/1 -> Regen_Disable/1
  Data Type Conversion3/1 -> Engine_On/1
  [VehSpdAvgDrvn] -> Veh_Spd/1
  Constant1/1 -> Conversion  APP1 (%)/1
  [PRNDL_Flt_ON] -> Switch1/2
  Switch3/1 -> 0 to 100%/1
  Override_APP/1 -> Switch3/2
  APP_value0_100/1 -> Switch3/1
  Key_Position/1 -> Switch4/3
  Override_KeyPos/1 -> Switch4/2
  KeyPos_value0_4/1 -> Switch4/1
  Switch4/1 -> Data Type Conversion/1
  Latch/1 -> Switch2/2
  Override_BPP/1 -> Switch5/2
  BPP_value0_100/1 -> Switch5/1
  Switch5/1 -> "0 to 100% "/1
  Override_PRNDL/1 -> Switch6/2
  PRNDL_value0_4/1 -> Switch6/1
  Switch6/1 -> Data Type Conversion1/1

== system HybridPowertrain_TestBench_Final/Driver/Manual Control ==
  note: Manipulate these values
      | to drive vehicle
  APP[%] : Constant
  BPP[%] : Constant  Value=-1
  Bus Creator1 : BusCreator  Inputs=5
  KeyPosition : Constant  Value=3
  PRNDL : Constant  Value=4
  ReferenceVel1 : Constant  Value=0
  Saturation : Saturate  UpperLimit=100  LowerLimit=0
  Saturation1 : Saturate  UpperLimit=0  LowerLimit=-100
  Saturation2 : Saturate  UpperLimit=3  LowerLimit=0
  Saturation3 : Saturate  UpperLimit=4  LowerLimit=0
  Slider Gain : simulink/Math Operations/Slider Gain  low=0  gain=1  high=2
  Slider Gain1 : simulink/Math Operations/Slider Gain  low=0  gain=1  high=2
  Out1 : Outport
  wires:
  Saturation2/1 -> Bus Creator1/3  "Key_Pos_[0_3]"
  Saturation1/1 -> Bus Creator1/2  "BPP(%)"
  Saturation/1 -> Bus Creator1/1  "APP (%)"
  KeyPosition/1 -> Saturation2/1
  Bus Creator1/1 -> Out1/1  "DriverOut"
  BPP[%]/1 -> Slider Gain1/1
  APP[%]/1 -> Slider Gain/1
  ReferenceVel1/1 -> Bus Creator1/5  "refVel [m/s]"
  PRNDL/1 -> Saturation3/1
  Saturation3/1 -> Bus Creator1/4  "PRNDL"
  Slider Gain/1 -> Saturation/1
  Slider Gain1/1 -> Saturation1/1

== system HybridPowertrain_TestBench_Final/Driver/Subsystem ==
  In1 : Inport
  Add1 : Sum  Inputs=+++
  Add2 : Sum
  Constant1 : Constant  Value=0
  Constant2 : Constant  Value=cal.APP.Mismatch_Value+0.1
  Constant3 : Constant  Value=0
  Constant4 : Constant  Value=cal.APP2.IN_Max_SC_Prcnt+1
  Constant5 : Constant  Value=0
  Constant6 : Constant  Value=cal.APP2.IN_Max_SC_Prcnt+1
  Switch : Switch  Threshold=1
  Switch1 : Switch  Threshold=1
  Switch2 : Switch  Threshold=1
  APP1 : Outport
  APP2 : Outport  Port=2
  wires:
  [Mismatch_APP_ON] -> Switch/2
  Switch/1 -> Add1/2
  Constant1/1 -> Switch/3
  Constant2/1 -> Switch/1
  Constant3/1 -> Switch1/3
  Constant4/1 -> Switch1/1
  [APP2_OOR_ON] -> Switch1/2
  Switch1/1 -> Add1/3
  Add1/1 -> APP2/1  "drv_APP2"
  In1/1 -> Add2/1, Add1/1
  Constant5/1 -> Switch2/3
  Constant6/1 -> Switch2/1
  [APP2_OOR_ON] -> Switch2/2
  Add2/1 -> APP1/1  "drv_APP1"
  Switch2/1 -> Add2/2
